simulink subsystem "subrMotorMechanics"  (R2024a)
settings: Solver=VariableStepAuto  StartTime=0.0  StopTime=10.0  RelTol=1e-3
model mask{J=J, B=B, D=D}
  mask prompts: J "Inertia"; B "Viscous Friction"; D "Coulomb Friction"
libraries: simulink x1
settings Model: Creator=anant  LastModifiedBy=anant

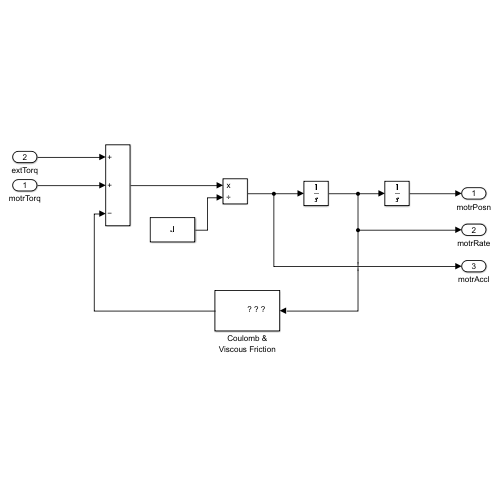
[thumbnail: Simulink's stored preview of the top-level diagram]
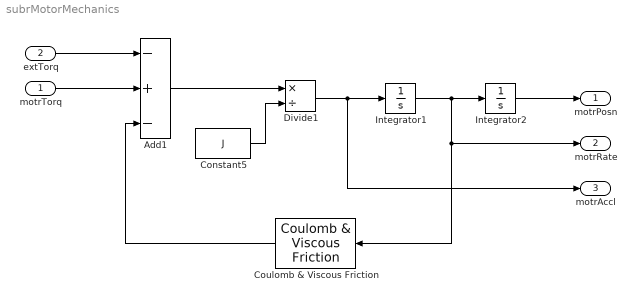
== system subrMotorMechanics ==
  motrTorq : Inport
  extTorq : Inport  Port=2
  Add1 : Sum  Inputs=-+-
  Constant5 : Constant  Value=J
  Coulomb & Viscous Friction : simulink/Discontinuities/Coulomb & Viscous Friction  offset=D  gain=B
  Divide1 : Product  Inputs=*/
  Integrator1 : Integrator
  Integrator2 : Integrator
  motrPosn : Outport
  motrRate : Outport  Port=2
  motrAccl : Outport  Port=3
  wires:
  Add1/1 -> Divide1/1
  Integrator1/1 -> motrRate/1, Coulomb & Viscous Friction/1, Integrator2/1
  Divide1/1 -> Integrator1/1, motrAccl/1
  Constant5/1 -> Divide1/2
  Integrator2/1 -> motrPosn/1
  extTorq/1 -> Add1/1
  motrTorq/1 -> Add1/2
  Coulomb & Viscous Friction/1 -> Add1/3
